simulink model "TaskA2"  (R2022b)
settings: Solver=VariableStepAuto  StartTime=0.0  StopTime=10.0  RelTol=1e-3
undefined symbols (not defined in the file): C, DiscIntNeverNeededParam, init, K_I2, K_x2
libraries: simulink_extras x4
settings Model: Creator=tumisangramotlhwa  LastModifiedBy=tumisangramotlhwa

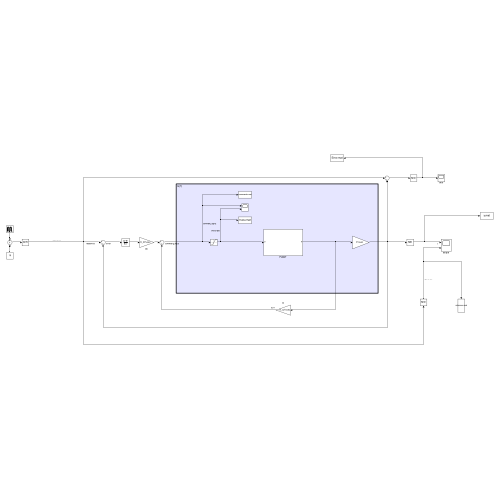
[thumbnail: Simulink's stored preview of the top-level diagram]
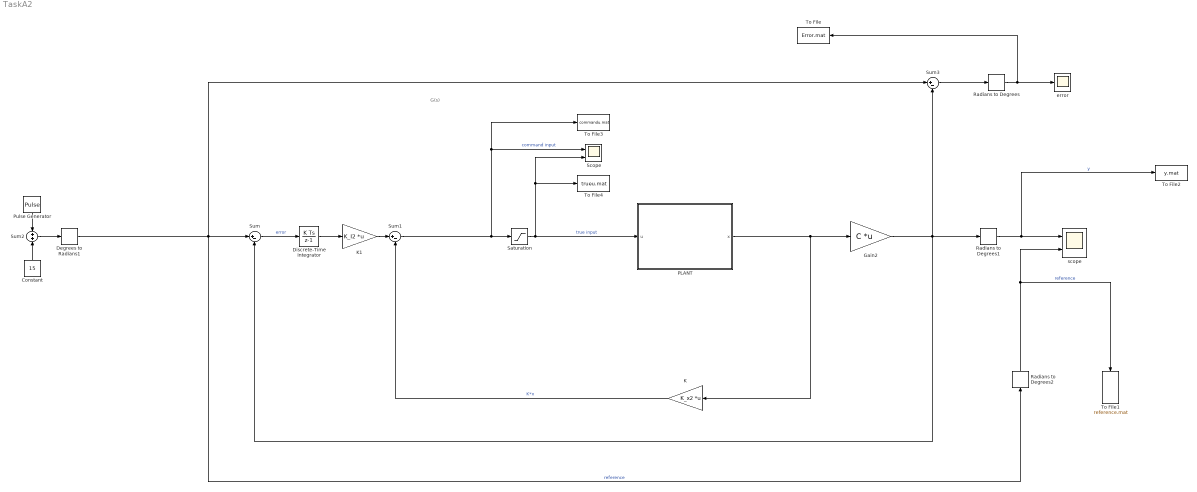
== system TaskA2 ==
  note: G(s)
  Constant : Constant  Value=15
  Degrees to Radians1 : simulink_extras/Transformations/Degrees to Radians
  Discrete-Time Integrator : DiscreteIntegrator  SampleTime=-1  ICPrevOutput=DiscIntNeverNeededParam  ICPrevScaledInput=DiscIntNeverNeededParam
  Gain2 : Gain  Gain=C  Multiplication=Matrix(K*u) (u vector)
  K : Gain  Gain=K_x2  Multiplication=Matrix(K*u) (u vector)
  K1 : Gain  Gain=K_I2  Multiplication=Matrix(K*u) (u vector)
  PLANT : Subsystem
  Pulse Generator : DiscretePulseGenerator  PulseType=Time based  Amplitude=30  Period=4  PulseWidth=50
  Radians to Degrees : simulink_extras/Transformations/Radians to Degrees
  Radians to Degrees1 : simulink_extras/Transformations/Radians to Degrees
  Radians to Degrees2 : simulink_extras/Transformations/Radians to Degrees
  Saturation : Saturate  UpperLimit=6  LowerLimit=-6
  Scope : Scope  NumInputPorts=2
  Sum : Sum  Inputs=|+-
  Sum1 : Sum  Inputs=|+-
  Sum2 : Sum  Inputs=+|+
  Sum3 : Sum  Inputs=|+-
  To File : ToFile  Filename=Error.mat  MatrixName=Error  SaveFormat=Timeseries
  To File1 : ToFile  Filename=reference.mat  MatrixName=reference  SaveFormat=Timeseries
  To File2 : ToFile  Filename=y.mat  MatrixName=y  SaveFormat=Timeseries
  To File3 : ToFile  Filename=commandu.mat  MatrixName=commandu  SaveFormat=Timeseries
  To File4 : ToFile  Filename=trueu.mat  MatrixName=trueu  SaveFormat=Timeseries
  error : Scope
  scope : Scope  NumInputPorts=2
  wires:
  Sum/1 -> Discrete-Time Integrator/1  "error"
  PLANT/1(x) -> Gain2/1, K/1
  Pulse Generator/1 -> Sum2/1
  Saturation/1 -> PLANT/1(u), To File4/1, Scope/2  "true input"
  Sum1/1 -> To File3/1, Scope/1, Saturation/1  "command input"
  Constant/1 -> Sum2/2
  Radians to Degrees2/1 -> scope/2, To File1/1  "reference"
  Radians to Degrees/1 -> error/1, To File/1
  Sum3/1 -> Radians to Degrees/1
  Gain2/1 -> Sum3/2, Sum/2, Radians to Degrees1/1
  K/1 -> Sum1/2  "K*x"
  Radians to Degrees1/1 -> To File2/1, scope/1  "y"
  Degrees to Radians1/1 -> Radians to Degrees2/1, Sum3/1, Sum/1  "reference"
  K1/1 -> Sum1/1
  Discrete-Time Integrator/1 -> K1/1
  Sum2/1 -> Degrees to Radians1/1

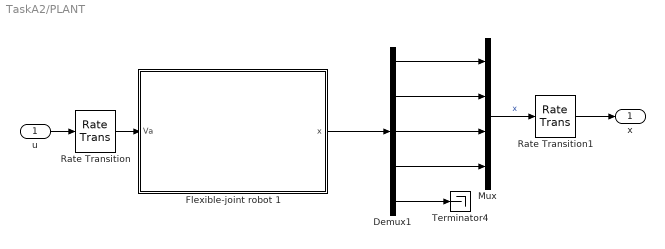
== system TaskA2/PLANT ==
  u : Inport
  Demux1 : Demux  Outputs=5
  Flexible-joint robot 1 : Subsystem
      mask Display: image('$imagefile'); % Use "Edit Image" on toolstrip to change.
  Mux : Mux
  Rate Transition : RateTransition  OutPortSampleTime=Ts
  Rate Transition1 : RateTransition  OutPortSampleTime=Ts
  Terminator4 : Terminator
  x : Outport
  wires:
  Mux/1 -> Rate Transition1/1  "x"
  Demux1/4 -> Mux/4
  Flexible-joint robot 1/1(x) -> Demux1/1
  Demux1/3 -> Mux/3
  Demux1/2 -> Mux/2
  Demux1/1 -> Mux/1
  Demux1/5 -> Terminator4/1
  u/1 -> Rate Transition/1
  Rate Transition/1 -> Flexible-joint robot 1/1(Va)
  Rate Transition1/1 -> x/1

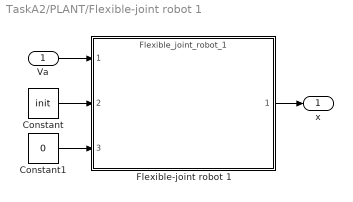
== system TaskA2/PLANT/Flexible-joint robot 1 ==
  Va : Inport
  Constant : Constant  Value=init
  Constant1 : Constant  Value=0
  Flexible-joint robot 1 : ModelReference  ModelNameDialog=Flexible_joint_robot_1  ModelReferenceVersion=1.63  CopyOfModelProtected=on
  x : Outport
  wires:
  Constant/1 -> Flexible-joint robot 1/2
  Constant1/1 -> Flexible-joint robot 1/3
  Flexible-joint robot 1/1 -> x/1
  Va/1 -> Flexible-joint robot 1/1
